simulink model "PMSM_control"  (R2018a)
settings: Solver=VariableStepAuto  StartTime=0.0  StopTime=50  FixedStep=0.0005  MaxStep=0.01
values from neighbouring files (symbols this model uses):
  b_eq = b_m + b_l/r^2    (= 1.5637748692e-05)    [PMSM_AyME.m]    (also in estabilidad_open_loop.m)
  ba = n*J_eq*w_pos    (= 0.0113019895361)    [PMSM_AyME.m]
  C_t = 1.091    [PMSM_AyME.m]
  J_eq = J_m + J_l/r^2    (= 5.65099476805e-06)    [PMSM_AyME.m]    (also in estabilidad_open_loop.m)
  K_e_omega = 3*p_obs^2    (= 30720000)    [PMSM_AyME.m]
  K_e_theta = -3*p_obs    (= 9600)    [PMSM_AyME.m]
  Ksa = n*J_eq*w_pos*w_pos    (= 9.04159162887)    [PMSM_AyME.m]
  Ksia = J_eq*w_pos*w_pos*w_pos    (= 2893.30932124)    [PMSM_AyME.m]
  L_d = 6.6E-3    (= 0.0066)    [PMSM_AyME.m]    (also in estabilidad_open_loop.m)
  L_q = 5.8E-3    (= 0.0058)    [PMSM_AyME.m]    (also in estabilidad_open_loop.m)
  lambda_m = 0.01546    [PMSM_AyME.m]    (also in estabilidad_open_loop.m)
  Lls = 0.8E-3    (= 0.0008)    [PMSM_AyME.m]    (also in estabilidad_open_loop.m)
  Pp = 3    [PMSM_AyME.m]    (also in estabilidad_open_loop.m)
  r = 314.3008    [PMSM_AyME.m]    (also in estabilidad_open_loop.m)
  R_0 = -p_i*Lls    (= 4)    [PMSM_AyME.m]
  R_d = -p_i*L_d    (= 33)    [PMSM_AyME.m]
  R_q = -p_i*L_q    (= 29)    [PMSM_AyME.m]
  R_s = 1.02    [PMSM_AyME.m]    (also in estabilidad_open_loop.m)
  R_tsa = 55    [PMSM_AyME.m]
  Tl = 1.57    [PMSM_AyME.m]    (also in estabilidad_open_loop.m)
undefined symbols (not defined in the file or in its folder): sigbuilder_block
libraries: dspsigops x3, peTransforms x1, simulink x1
settings Model: PacingRate=1000  Creator=gino  LastModifiedBy=gino
settings SolverCC: ZeroCrossControl=EnableAll

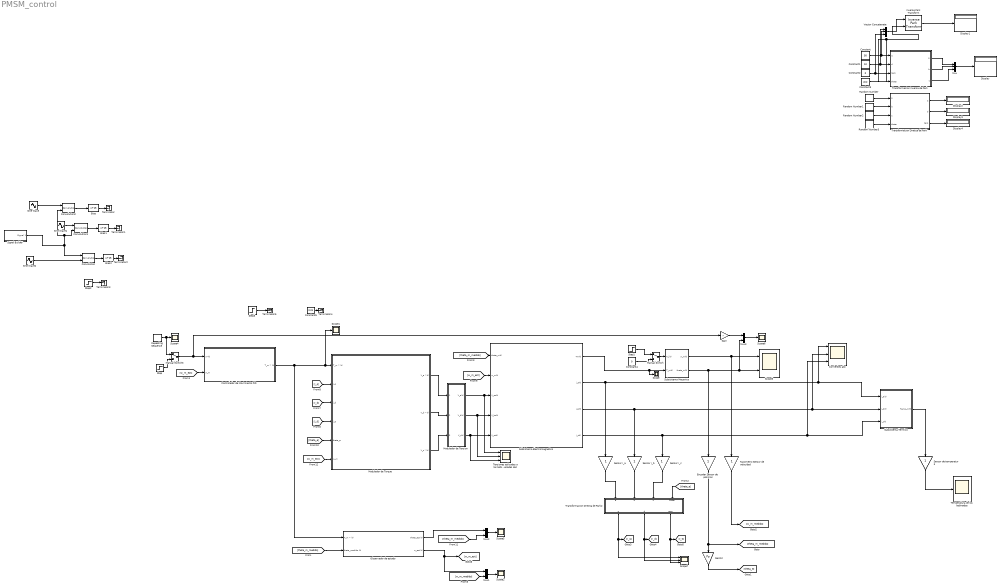
== system PMSM_control ==
  Bias : Bias  Bias=15
  Bias1 : Bias  Bias=15
  Bias2 : Bias  Bias=15
  Constant : Constant  Value=50
  Constant1 : Constant  Value=10
  Constant2 : Constant  Value=0
  Constant3 : Constant  Value=pi/2
  Constant4 : Constant  Value=0
  Constant5 : Constant  Value=0.01
  Controlador de Movimiento PID : Subsystem
  Convolution : dspsigops/Convolution  domain=Time  roundingMode=Floor  overflowMode=off  outputDataTypeStr=Inherit: Same as accumulator  outputMin=[]  outputMax=[]  outputLastDataTypeStr=Inherit: Same as accumulator
      settings: SourceProductName=DSP System Toolbox  SourceProductBaseCode=DS
  Convolution1 : dspsigops/Convolution  domain=Time  roundingMode=Floor  overflowMode=off  outputDataTypeStr=Inherit: Same as accumulator  outputMin=[]  outputMax=[]  outputLastDataTypeStr=Inherit: Same as accumulator
      settings: SourceProductName=DSP System Toolbox  SourceProductBaseCode=DS
  Convolution2 : dspsigops/Convolution  domain=Time  roundingMode=Floor  overflowMode=off  outputDataTypeStr=Inherit: Same as accumulator  outputMin=[]  outputMax=[]  outputLastDataTypeStr=Inherit: Same as accumulator
      settings: SourceProductName=DSP System Toolbox  SourceProductBaseCode=DS
  Corrientes abc : Scope  NumInputPorts=3
  Display{,1..4} (5 alike) : Display
  Encoder Sensor de posicion : Gain
  Gain : Gain  Gain=r
  Gain12 : Gain  Gain=Pp
  Inverse Park Transform : peTransforms/Inverse Park Transform  AxisAlignment=Q-axis  PowerInvariant=off
  Manual Switch : ManualSwitch
  Manual Switch3 : ManualSwitch
  Modulador de Tension : Subsystem
  Modulador de Torque : Subsystem
  Mux : Mux  Inputs=3
  Mux1 : Mux  Inputs=2
  Mux2 : Mux  Inputs=2
  Mux3 : Mux  Inputs=2
  Observador de estado : Subsystem
  Random Number{,1..3} (4 alike) : RandomNumber  SampleTime=0.1
  Repeating Sequence : simulink/Sources/Repeating Sequence  rep_seq_t=[0 5 10 15 20 25 30 35 40]  rep_seq_y="[0 0 2*pi 2*pi 0 0  -2*pi -2*pi 0]"
  Scope{,1..2,4..6} (6 alike) : Scope
  Scope3 : Scope  NumInputPorts=2
  Scope7 : Scope  NumInputPorts=3
  Sensor de temperatura : Gain
  Sensor i_a : Gain
  Sensor i_b : Gain
  Sensor i_c : Gain
  Signal Builder : Subsystem  Tag=STV Subsys  LoadFcn=sigbuilder_block('load');  StartFcn=sigbuilder_block('start');  StopFcn=sigbuilder_block('stop');  ClipboardFcn=sigbuilder_block('clipboard');  mask(Sigbuilder block){tuvar=[0:10]}
      mask help: Simulink:masks:SigbuilderBlock_MD
      mask init:
      | if ~strcmp(get_param(bdroot(gcbh),'SimulationStatus'),'stopped') tuvar = sigbuilder_block('maskInit'); end
      settings: CopyFcn=sigbuilder_block('copy');  DeleteFcn=sigbuilder_block('delete');  ModelCloseFcn=sigbuilder_block('modelClose');  PreSaveFcn=sigbuilder_block('preSave');  PauseFcn=sigbuilder_block('pause');  ContinueFcn=sigbuilder_block('continue');  NameChangeFcn=sigbuilder_block('namechange');  OpenFcn=sigbuilder_block('open',[242.25 102.75 550.5 357 ]);  CloseFcn=sigbuilder_block('close');
      mask Display: plot(0, 0, 100, 100,[2, 2, 32, 32, 2], [68, 8, 8, 68, 68],[32, 2], [38, 38], [32, 19, 2],[53, 60, 44], [32, 17, 17, 2],[16, 16, 31, 31]);txt = getActiveGroup(gcbh);text(2, 100, txt,'verticalAlignment', 'top');
  Sine Wave : Sin  Amplitude=30  Frequency=300*2*pi  SampleTime=0
  Sine Wave1 : Sin  Amplitude=30  Frequency=300*2*pi  Phase=2*pi/3  SampleTime=0
  Sine Wave2 : Sin  Amplitude=30  Frequency=300*2*pi  Phase=4*pi/3  SampleTime=0
  Step : Step  After=0.1  SampleTime=0
  Step1 : Step  Time=0.3  After=Tl  SampleTime=0
  Step2 : Step  Time=0.1  After=19.596  SampleTime=0
  Step3 : Step  Time=0.1  After=0.001  SampleTime=0
  Subsistema Electromagnetico : Subsystem
  Subsistema Mecanico : Subsystem
  Subsistema Termico : Subsystem
  Tacometro Sensor de velocidad : Gain
  Temperatura de los bobinados : Scope
  Tensiones aplicadas a los bobinados en coordenadas abc : Scope  NumInputPorts=3
  Terminator{,1..5} (6 alike) : Terminator
  Transformacion Directa de Park : MATLAB Function  TreatAsAtomicUnit=on
  Transformacion Directa de Park2 : MATLAB Function  TreatAsAtomicUnit=on
  Transformacion Inversa de Park : MATLAB Function  TreatAsAtomicUnit=on
  Vector Concatenate : Concatenate  NumInputs=3
  wires:
  Constant3/1 -> Inverse Park Transform/2, Transformacion Inversa de Park/4(theta)
  Constant2/1 -> Vector Concatenate/3, Transformacion Inversa de Park/3(zero)
  Constant1/1 -> Vector Concatenate/1, Transformacion Inversa de Park/2(d)
  Constant/1 -> Vector Concatenate/2, Transformacion Inversa de Park/1(q)
  Transformacion Inversa de Park/2(b) -> Mux/2
  Transformacion Inversa de Park/1(a) -> Mux/1
  Transformacion Inversa de Park/3(c) -> Mux/3
  Mux/1 -> Display/1
  Vector Concatenate/1 -> Inverse Park Transform/1
  Inverse Park Transform/1 -> Display1/1
  Manual Switch/1 -> Subsistema Mecanico/1(T_l(t))
  Constant4/1 -> Manual Switch/2
  Convolution1/1 -> Bias1/1
  Signal Builder/1(Signal 1) -> Convolution/1, Convolution1/2, Convolution2/2
  Sine Wave2/1 -> Convolution/2
  Sine Wave1/1 -> Convolution1/1
  Sine Wave/1 -> Convolution2/1
  Convolution/1 -> Bias2/1
  Convolution2/1 -> Bias/1
  Random Number2/1 -> Transformacion Directa de Park/3(c)
  Random Number3/1 -> Transformacion Directa de Park/4(theta)
  Random Number1/1 -> Transformacion Directa de Park/2(b)
  Random Number/1 -> Transformacion Directa de Park/1(a)
  Transformacion Directa de Park/3(zero) -> Display4/1
  Transformacion Directa de Park/2(d) -> Display3/1
  Transformacion Directa de Park/1(q) -> Display2/1
  Step1/1 -> Manual Switch/1
  Transformacion Directa de Park2/2(d) -> Scope7/2, [i_d]
  Transformacion Directa de Park2/3(zero) -> [i_0], Scope7/3
  Subsistema Electromagnetico/1(Tm(t)) -> Scope/1, Subsistema Mecanico/2(T_m(t))
  Subsistema Mecanico/2(theta_m(t)) -> Mux3/2, Scope3/2, Encoder Sensor de posicion/1
  Modulador de Tension/3(V_c(t)) -> Subsistema Electromagnetico/5(V_cs(t)), Tensiones aplicadas a los bobinados en coordenadas abc/3
  Modulador de Tension/2(V_b(t)) -> Subsistema Electromagnetico/4(V_bs(t)), Tensiones aplicadas a los bobinados en coordenadas abc/2
  Modulador de Tension/1(V_a(t)) -> Tensiones aplicadas a los bobinados en coordenadas abc/1, Subsistema Electromagnetico/3(V_as(t))
  Transformacion Directa de Park2/1(q) -> [i_q], Scope7/1
  Subsistema Mecanico/1(w_m(t)) -> Scope3/1, Tacometro Sensor de velocidad/1
  Subsistema Electromagnetico/2(i_a(t)) -> Sensor i_a/1, Corrientes abc/1, Subsistema Termico/1(i_a(t))
  Subsistema Termico/1(Temp_m(t)) -> Sensor de temperatura/1
  Subsistema Electromagnetico/3(i_b(t)) -> Subsistema Termico/2(i_b(t)), Corrientes abc/2, Sensor i_b/1
  Sensor de temperatura/1 -> Temperatura de los bobinados/1
  Subsistema Electromagnetico/4(i_c(t)) -> Corrientes abc/3, Subsistema Termico/3(i_c(t)), Sensor i_c/1
  Gain12/1 -> [theta_e]
  [theta_m_medido] -> Subsistema Electromagnetico/1("theta_m(t) ")
  [theta_e] -> Transformacion Directa de Park2/4(theta)
  Encoder Sensor de posicion/1 -> Gain12/1, [theta_m_medido]
  Sensor i_b/1 -> Transformacion Directa de Park2/2(b)
  Sensor i_a/1 -> Transformacion Directa de Park2/1(a)
  Sensor i_c/1 -> Transformacion Directa de Park2/3(c)
  Tacometro Sensor de velocidad/1 -> [w_m_medido]
  [w_m_est] -> Subsistema Electromagnetico/2(w_m(t))
  Bias/1 -> Terminator/1
  Bias1/1 -> Terminator1/1
  Bias2/1 -> Terminator2/1
  Step2/1 -> Terminator3/1
  Constant5/1 -> Terminator4/1
  [w_m_est] -> Modulador de Torque/6("w_m ")
  [theta_e] -> Modulador de Torque/5(theta_e)
  [i_0] -> Modulador de Torque/4(i_0)
  [i_d] -> Modulador de Torque/3(i_d)
  [i_q] -> Modulador de Torque/2(i_q)
  Modulador de Torque/3(V_c * (t)) -> Modulador de Tension/3(V_c * (t))
  Modulador de Torque/2(V_b * (t)) -> Modulador de Tension/2(V_b * (t))
  Modulador de Torque/1(V_a * (t)) -> Modulador de Tension/1(V_a * (t))
  Controlador de Movimiento PID/1(T_m *' (t)) -> Scope1/1, Modulador de Torque/1(T_m *' (t)), Observador de estado/1(T_m *' (t))
  Repeating Sequence/1 -> Manual Switch3/1, Scope4/1
  Step/1 -> Manual Switch3/2
  Manual Switch3/1 -> Gain/1, Controlador de Movimiento PID/1(w*(t))
  [w_m_est] -> Controlador de Movimiento PID/2(w_m)
  [theta_m_medido] -> Observador de estado/2(theta_medido (t))
  [w_m_medido] -> Mux1/2
  Observador de estado/2(w_est (t)) -> Mux1/1, [w_m_est]
  Mux1/1 -> Scope2/1
  Mux2/1 -> Scope5/1
  [theta_m_medido] -> Mux2/2
  Observador de estado/1(theta_est (t)) -> Mux2/1
  Step3/1 -> Terminator5/1
  Mux3/1 -> Scope6/1
  Gain/1 -> Mux3/1

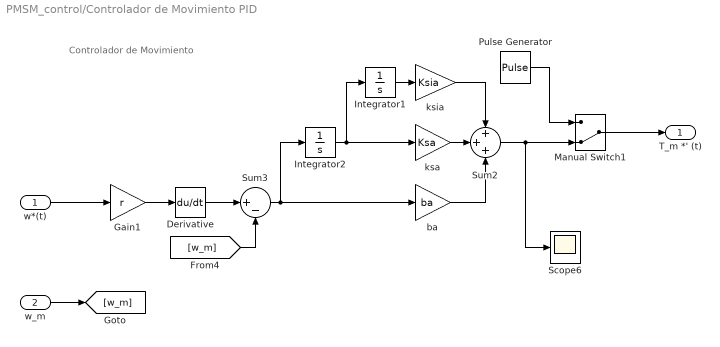
== system PMSM_control/Controlador de Movimiento PID ==
  note: Controlador de Movimiento
  w*(t) : Inport
  w_m : Inport  Port=2
  Derivative : Derivative
  Gain1 : Gain  Gain=r
  Integrator1 : Integrator
  Integrator2 : Integrator
  Manual Switch1 : ManualSwitch  CurrentSetting=0
  Pulse Generator : DiscretePulseGenerator  PulseType=Time based  Amplitude=0.001  Period=1
  Scope6 : Scope
  Sum2 : Sum  Inputs=+++
  Sum3 : Sum  Inputs=|+-
  ba : Gain  Gain=ba
  "ksa " : Gain  Gain=Ksa
  "ksia " : Gain  Gain=Ksia
  T_m *' (t) : Outport
  wires:
  "ksia "/1 -> Sum2/1
  "ksa "/1 -> Sum2/2
  [w_m] -> Sum3/2
  Sum2/1 -> Manual Switch1/2, Scope6/1
  Pulse Generator/1 -> Manual Switch1/1
  Gain1/1 -> Derivative/1
  Integrator2/1 -> "ksa "/1, Integrator1/1
  Integrator1/1 -> "ksia "/1
  Manual Switch1/1 -> T_m *' (t)/1
  Derivative/1 -> Sum3/1
  Sum3/1 -> ba/1, Integrator2/1
  ba/1 -> Sum2/3
  w*(t)/1 -> Gain1/1
  w_m/1 -> [w_m]

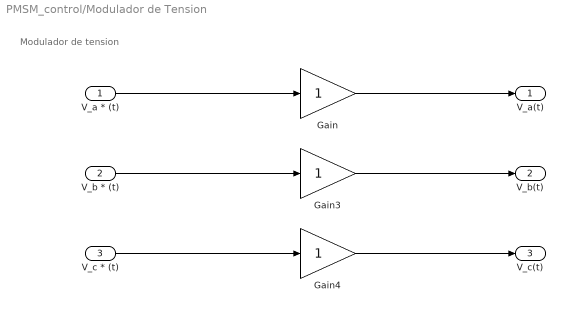
== system PMSM_control/Modulador de Tension ==
  note: Modulador de tension
  V_a * (t) : Inport
  V_b * (t) : Inport  Port=2
  V_c * (t) : Inport  Port=3
  Gain : Gain
  Gain3 : Gain
  Gain4 : Gain
  V_a(t) : Outport
  V_b(t) : Outport  Port=2
  V_c(t) : Outport  Port=3
  wires:
  V_a * (t)/1 -> Gain/1
  Gain/1 -> V_a(t)/1
  V_b * (t)/1 -> Gain3/1
  V_c * (t)/1 -> Gain4/1
  Gain3/1 -> V_b(t)/1
  Gain4/1 -> V_c(t)/1

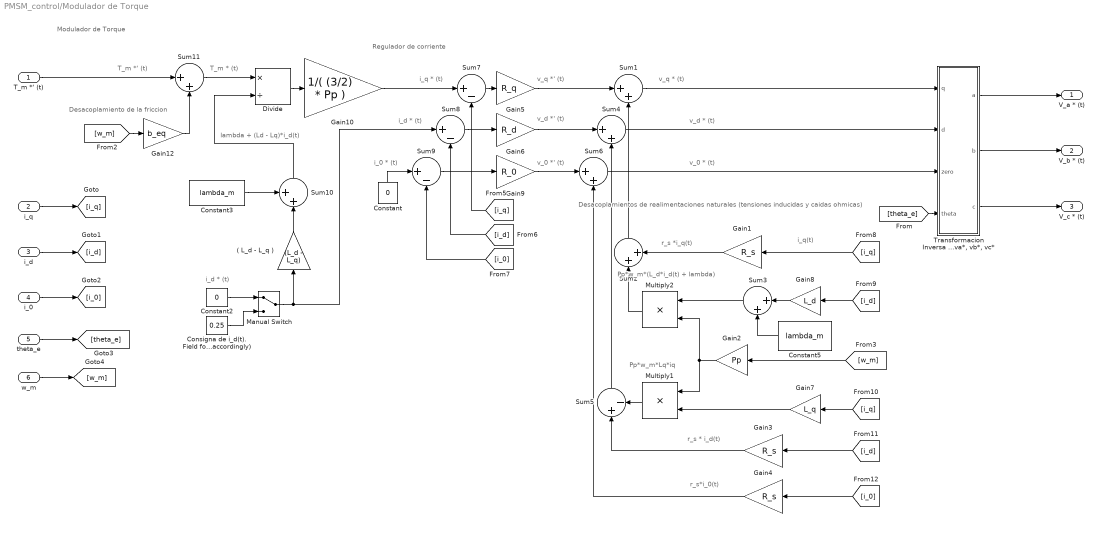
== system PMSM_control/Modulador de Torque ==
  note: lambda + (Ld - Lq)*i_d(t)
  note: Modulador de Torque
  note: T_m *' (t)
  note: Regulador de corriente
  note: Desacoplamiento de la friccion
  note: T_m * (t)
  note: i_d * (t)
  note: i_0 * (t)
  note: i_q * (t)
  note: i_d * (t)
  note: Desacoplamientos de realimentaciones naturales
      | (tensiones inducidas y caidas ohmicas)
  note: v_0 * (t)
  note: v_d * (t)
  note: r_s*i_0(t)
  note: Pp*w_m*Lq*iq
  note: r_s * i_d(t)
  note: Pp*w_m*(L_d*i_d(t) + lambda)
  note: r_s *i_q(t)
  note: v_q * (t)
  note: i_q(t)
  note: v_q *' (t)
  note: v_d *' (t)
  note: v_0 *' (t)
  T_m *' (t) : Inport
  i_q : Inport  Port=2
  i_d : Inport  Port=3
  i_0 : Inport  Port=4
  theta_e : Inport  Port=5
  "w_m " : Inport  Port=6
  ( L_d - L_q ) : Gain  Gain=(L_d - L_q)
  Consigna de i_d(t). Field forcing or weakening (change sign accordingly) : Constant  Value=0.25
  Constant : Constant  Value=0
  Constant2 : Constant  Value=0
  Constant3 : Constant  Value=lambda_m
  Constant5 : Constant  Value=lambda_m
  Divide : Product  Inputs=*/
  Gain1 : Gain  Gain=R_s
  Gain10 : Gain  Gain=1/( (3/2) * Pp )
  Gain12 : Gain  Gain=b_eq
  Gain2 : Gain  Gain=Pp
  Gain3 : Gain  Gain=R_s
  Gain4 : Gain  Gain=R_s
  Gain5 : Gain  Gain=R_q
  Gain6 : Gain  Gain=R_d
  Gain7 : Gain  Gain=L_q
  Gain8 : Gain  Gain=L_d
  Gain9 : Gain  Gain=R_0
  Manual Switch : ManualSwitch
  Multiply1 : Product
  Multiply2 : Product
  Sum{1..4,6,11} (6 alike) : Sum  Inputs=|++
  Sum10 : Sum  Inputs=++|
  Sum{5,7..9} (4 alike) : Sum  Inputs=|+-
  "Transformacion Inversa de Park vq*, vd*, v0* --> va*, vb*, vc*" : MATLAB Function  TreatAsAtomicUnit=on
  V_a * (t) : Outport
  V_b * (t) : Outport  Port=2
  V_c * (t) : Outport  Port=3
  wires:
  Gain7/1 -> Multiply1/2
  [i_q] -> Sum7/2
  Gain5/1 -> Sum1/1
  Sum9/1 -> Gain9/1
  Sum8/1 -> Gain6/1
  Constant5/1 -> Sum3/2
  Sum1/1 -> "Transformacion Inversa de Park vq*, vd*, v0* --> va*, vb*, vc*"/1(q)
  Constant/1 -> Sum9/1
  Sum5/1 -> Sum4/2
  [i_q] -> Gain1/1
  Sum3/1 -> Multiply2/1
  Gain1/1 -> Sum2/2
  [i_0] -> Gain4/1
  Gain2/1 -> Multiply1/1, Multiply2/2
  [i_q] -> Gain7/1
  [i_d] -> Gain3/1
  Sum2/1 -> Sum1/2
  [theta_e] -> "Transformacion Inversa de Park vq*, vd*, v0* --> va*, vb*, vc*"/4(theta)
  Sum6/1 -> "Transformacion Inversa de Park vq*, vd*, v0* --> va*, vb*, vc*"/3(zero)
  Sum4/1 -> "Transformacion Inversa de Park vq*, vd*, v0* --> va*, vb*, vc*"/2(d)
  [i_d] -> Sum8/2
  [i_d] -> Gain8/1
  Gain3/1 -> Sum5/1
  Gain9/1 -> Sum6/1
  [i_0] -> Sum9/2
  Multiply1/1 -> Sum5/2
  Gain6/1 -> Sum4/1
  Sum7/1 -> Gain5/1
  Multiply2/1 -> Sum2/1
  Gain8/1 -> Sum3/1
  Gain4/1 -> Sum6/2
  [w_m] -> Gain2/1
  Constant2/1 -> Manual Switch/1
  Consigna de i_d(t). Field forcing or weakening (change sign accordingly)/1 -> Manual Switch/2
  Gain10/1 -> Sum7/1
  Divide/1 -> Gain10/1
  Constant3/1 -> Sum10/1
  ( L_d - L_q )/1 -> Sum10/2
  Sum10/1 -> Divide/2
  [w_m] -> Gain12/1
  Sum11/1 -> Divide/1
  theta_e/1 -> [theta_e]
  i_q/1 -> [i_q]
  i_0/1 -> [i_0]
  "w_m "/1 -> [w_m]
  i_d/1 -> [i_d]
  T_m *' (t)/1 -> Sum11/1
  Gain12/1 -> Sum11/2
  "Transformacion Inversa de Park vq*, vd*, v0* --> va*, vb*, vc*"/3(c) -> V_c * (t)/1
  "Transformacion Inversa de Park vq*, vd*, v0* --> va*, vb*, vc*"/2(b) -> V_b * (t)/1
  "Transformacion Inversa de Park vq*, vd*, v0* --> va*, vb*, vc*"/1(a) -> V_a * (t)/1
  Manual Switch/1 -> Sum8/1, ( L_d - L_q )/1

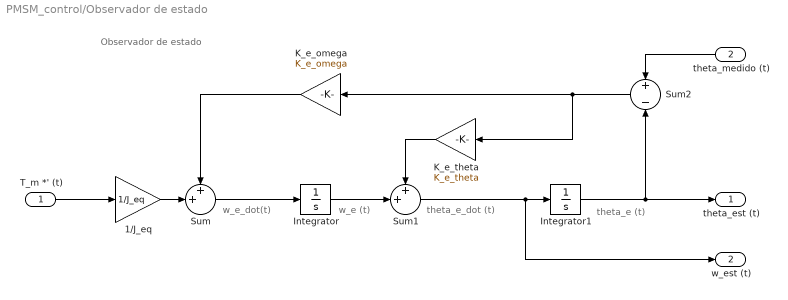
== system PMSM_control/Observador de estado ==
  note: Observador de estado
  note: theta_e (t)
  note: theta_e_dot (t)
  note: w_e (t)
  note: w_e_dot(t)
  T_m *' (t) : Inport
  theta_medido (t) : Inport  Port=2
  1/J_eq : Gain  Gain=1/J_eq
  Integrator : Integrator
  Integrator1 : Integrator
  K_e_omega : Gain  Gain=K_e_omega
  K_e_theta : Gain  Gain=K_e_theta
  Sum : Sum  Inputs=++|
  Sum1 : Sum  Inputs=++|
  Sum2 : Sum  Inputs=+-
  theta_est (t) : Outport
  w_est (t) : Outport  Port=2
  wires:
  Integrator1/1 -> theta_est (t)/1, Sum2/2
  Sum/1 -> Integrator/1
  T_m *' (t)/1 -> 1/J_eq/1
  1/J_eq/1 -> Sum/2
  K_e_omega/1 -> Sum/1
  Integrator/1 -> Sum1/2
  K_e_theta/1 -> Sum1/1
  Sum1/1 -> w_est (t)/1, Integrator1/1
  theta_medido (t)/1 -> Sum2/1
  Sum2/1 -> K_e_theta/1, K_e_omega/1

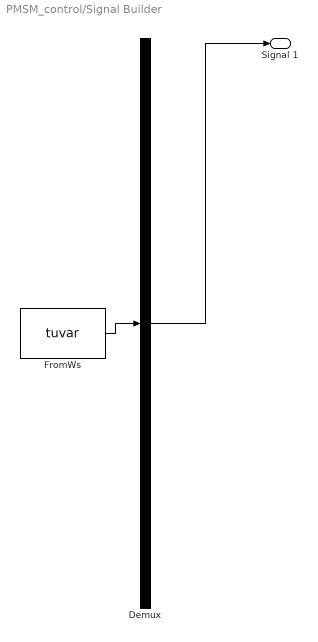
== system PMSM_control/Signal Builder ==
  Demux : Demux  Tag=STV Demux  Outputs=1
  FromWs : FromWorkspace  Tag=STV FromWs  VariableName=tuvar  SampleTime=0
      SigBuilderData=|
      | common.afterFinalStr = 'Extrapolate'
      | common.sampleTime = 0
      | dataSet.timeRange = [0 10]
      | dataSet.name = 'Group 1'
      | sbobj.Groups.Name = 'Group 1'
      | sbobj.Groups.Signals.Name = 'Signal 1'
      | sbobj.Groups.Signals.XData = [0 0.49 10]
      | sbobj.Groups.Signals.YData = [0 1 1]
  Signal 1 : Outport  Tag=STV Outport
  wires:
  Demux/1 -> Signal 1/1
  FromWs/1 -> Demux/1

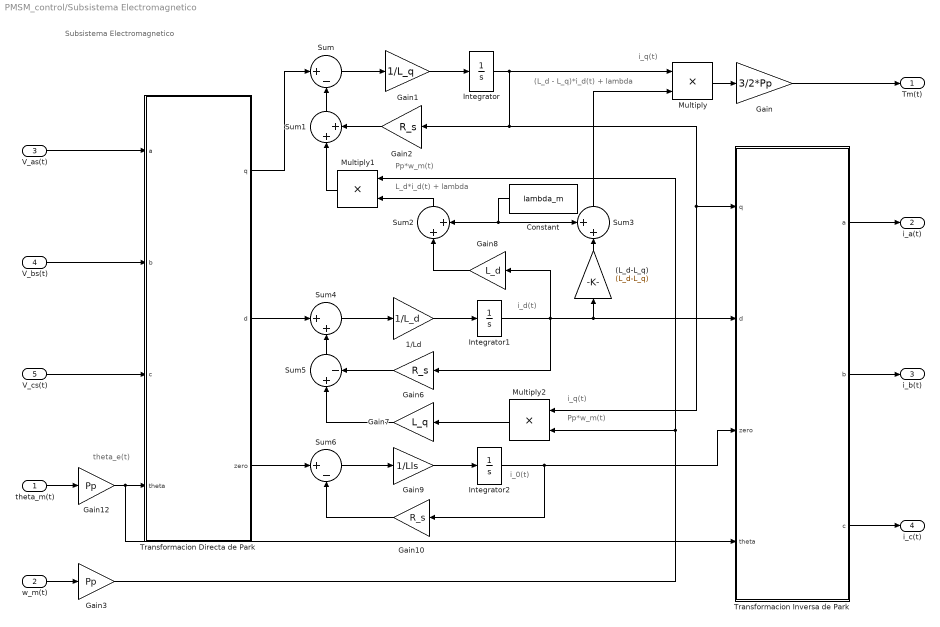
== system PMSM_control/Subsistema Electromagnetico ==
  note: Subsistema Electromagnetico
  note: (L_d - L_q)*i_d(t) + lambda
  note: L_d*i_d(t) + lambda
  note: theta_e(t)
  note: i_0(t)
  note: Pp*w_m(t)
  note: Pp*w_m(t)
  note: i_q(t)
  note: i_d(t)
  note: i_q(t)
  "theta_m(t) " : Inport
  w_m(t) : Inport  Port=2
  V_as(t) : Inport  Port=3
  V_bs(t) : Inport  Port=4
  V_cs(t) : Inport  Port=5
  (L_d-L_q) : Gain  Gain=(L_d-L_q)
  1/Ld : Gain  Gain=1/L_d
  Constant : Constant  Value=lambda_m
  Gain : Gain  Gain=3/2*Pp
  Gain1 : Gain  Gain=1/L_q
  Gain10 : Gain  Gain=R_s
  Gain12 : Gain  Gain=Pp
  Gain2 : Gain  Gain=R_s
  Gain3 : Gain  Gain=Pp
  Gain6 : Gain  Gain=R_s
  Gain7 : Gain  Gain=L_q
  Gain8 : Gain  Gain=L_d
  Gain9 : Gain  Gain=1/Lls
  Integrator : Integrator
  Integrator1 : Integrator
  Integrator2 : Integrator
  Multiply : Product
  Multiply1 : Product
  Multiply2 : Product
  Sum : Sum  Inputs=|+-
  Sum1 : Sum  Inputs=|++
  Sum2 : Sum  Inputs=|++
  Sum3 : Sum  Inputs=++|
  Sum4 : Sum  Inputs=|++
  Sum5 : Sum  Inputs=|+-
  Sum6 : Sum  Inputs=|+-
  Transformacion Directa de Park : MATLAB Function  TreatAsAtomicUnit=on
  Transformacion Inversa de Park : MATLAB Function  TreatAsAtomicUnit=on
  Tm(t) : Outport
  i_a(t) : Outport  Port=2
  i_b(t) : Outport  Port=3
  i_c(t) : Outport  Port=4
  wires:
  Gain/1 -> Tm(t)/1
  Multiply/1 -> Gain/1
  Integrator/1 -> Multiply/1, Transformacion Inversa de Park/1(q), Multiply2/1, Gain2/1
  Gain1/1 -> Integrator/1
  Sum/1 -> Gain1/1
  Sum1/1 -> Sum/2
  Gain2/1 -> Sum1/2
  Multiply1/1 -> Sum1/1
  w_m(t)/1 -> Gain3/1
  Gain3/1 -> Multiply1/1, Multiply2/2
  Sum3/1 -> Multiply/2
  Constant/1 -> Sum3/1, Sum2/2
  (L_d-L_q)/1 -> Sum3/2
  Integrator1/1 -> Gain6/1, Transformacion Inversa de Park/2(d), (L_d-L_q)/1, Gain8/1
  1/Ld/1 -> Integrator1/1
  Sum4/1 -> 1/Ld/1
  Gain6/1 -> Sum5/2
  Gain7/1 -> Sum5/1
  Multiply2/1 -> Gain7/1
  Gain8/1 -> Sum2/1
  Sum5/1 -> Sum4/2
  Transformacion Directa de Park/1(q) -> Sum/1
  Transformacion Directa de Park/2(d) -> Sum4/1
  Gain9/1 -> Integrator2/1
  Sum6/1 -> Gain9/1
  Gain10/1 -> Sum6/2
  Integrator2/1 -> Gain10/1, Transformacion Inversa de Park/3(zero)
  Transformacion Directa de Park/3(zero) -> Sum6/1
  "theta_m(t) "/1 -> Gain12/1
  Gain12/1 -> Transformacion Directa de Park/4(theta), Transformacion Inversa de Park/4(theta)
  V_as(t)/1 -> Transformacion Directa de Park/1(a)
  V_bs(t)/1 -> Transformacion Directa de Park/2(b)
  V_cs(t)/1 -> Transformacion Directa de Park/3(c)
  Transformacion Inversa de Park/1(a) -> i_a(t)/1
  Transformacion Inversa de Park/2(b) -> i_b(t)/1
  Transformacion Inversa de Park/3(c) -> i_c(t)/1
  Sum2/1 -> Multiply1/2

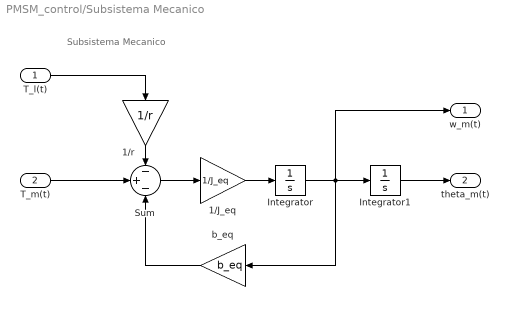
== system PMSM_control/Subsistema Mecanico ==
  note: Subsistema Mecanico
  T_l(t) : Inport
  T_m(t) : Inport  Port=2
  1/J_eq : Gain  Gain=1/J_eq
  1/r : Gain  Gain=1/r
  Integrator : Integrator
  Integrator1 : Integrator
  Sum : Sum  Inputs=-+-
  b_eq : Gain  Gain=b_eq
  w_m(t) : Outport
  theta_m(t) : Outport  Port=2
  wires:
  1/J_eq/1 -> Integrator/1
  Integrator1/1 -> theta_m(t)/1
  Integrator/1 -> Integrator1/1, w_m(t)/1, b_eq/1
  Sum/1 -> 1/J_eq/1
  T_l(t)/1 -> 1/r/1
  b_eq/1 -> Sum/3
  T_m(t)/1 -> Sum/2
  1/r/1 -> Sum/1

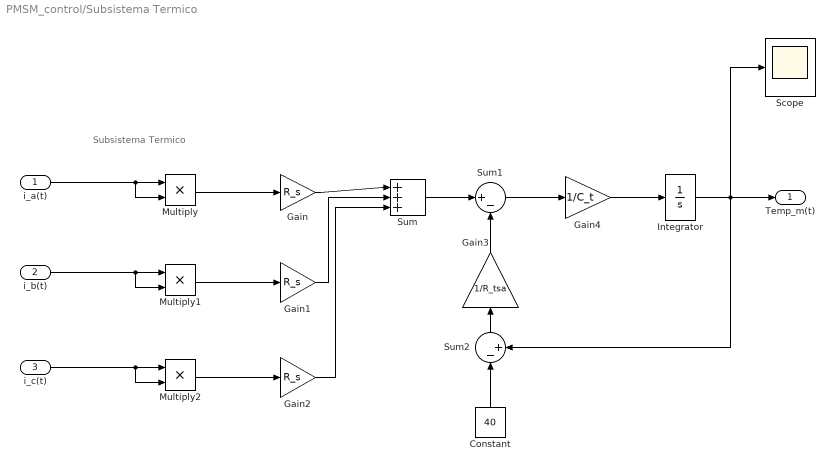
== system PMSM_control/Subsistema Termico ==
  note: Subsistema Termico
  i_a(t) : Inport
  i_b(t) : Inport  Port=2
  i_c(t) : Inport  Port=3
  Constant : Constant  Value=40
  Gain : Gain  Gain=R_s
  Gain1 : Gain  Gain=R_s
  Gain2 : Gain  Gain=R_s
  Gain3 : Gain  Gain=1/R_tsa
  Gain4 : Gain  Gain=1/C_t
  Integrator : Integrator  InitialCondition=40
  Multiply : Product
  Multiply1 : Product
  Multiply2 : Product
  Scope : Scope
  Sum : Sum  Inputs=|+++
  Sum1 : Sum  Inputs=|+-
  Sum2 : Sum  Inputs=|-+
  Temp_m(t) : Outport
  wires:
  i_a(t)/1 -> Multiply/1, Multiply/2
  i_b(t)/1 -> Multiply1/2, Multiply1/1
  i_c(t)/1 -> Multiply2/2, Multiply2/1
  Multiply/1 -> Gain/1
  Multiply1/1 -> Gain1/1
  Multiply2/1 -> Gain2/1
  Gain1/1 -> Sum/2
  Gain/1 -> Sum/1
  Gain2/1 -> Sum/3
  Sum/1 -> Sum1/1
  Gain3/1 -> Sum1/2
  Sum2/1 -> Gain3/1
  Constant/1 -> Sum2/1
  Sum1/1 -> Gain4/1
  Gain4/1 -> Integrator/1
  Integrator/1 -> Sum2/2, Temp_m(t)/1, Scope/1

== matlab function PMSM_control/Transformacion Inversa de Park ==
  data: q input; a output; d input; zero input; theta input; b output; c output
function [a, b, c] = inverse_park_transformation(q, d, zero, theta)
%Transformación inversa de Park
 
abc = [cos(theta)               sin(theta)              1
        cos(theta - 2*pi/3)     sin(theta - 2*pi/3)     1
        cos(theta + 2*pi/3)     sin(theta + 2*pi/3)     1] ...
    *   [q
        d
        zero];

a = abc(1);
b = abc(2);
c = abc(3);

end

== matlab function PMSM_control/Transformacion Directa de Park ==
  data: a input; q output; b input; c input; theta input; d output; zero output
function [q, d, zero] = park_transformation(a, b, c, theta)
%Transformación directa de Park
 
qdz = 2/3 * [cos(theta)     cos(theta - 2*pi/3)     cos(theta + 2*pi/3)
                    sin(theta)      sin(theta - 2*pi/3)     sin(theta + 2*pi/3)
                    1/2             1/2                     1/2] ...
                *   [a
                    b 
                    c];

q = qdz(1);
d = qdz(2);
zero = qdz(3);

end

== matlab function PMSM_control/Subsistema Electromagnetico/Transformacion Directa de Park ==
  data: a input; q output; b input; c input; theta input; d output; zero output
function [q, d, zero] = park_transformation(a, b, c, theta)
%Transformación directa de Park
 
qdz = 2/3 * [cos(theta)     cos(theta - 2*pi/3)     cos(theta + 2*pi/3)
                    sin(theta)      sin(theta - 2*pi/3)     sin(theta + 2*pi/3)
                    1/2             1/2                     1/2] ...
                *   [a
                    b 
                    c];

q = qdz(1);
d = qdz(2);
zero = qdz(3);

end

== matlab function PMSM_control/Subsistema Electromagnetico/Transformacion Inversa de Park ==
  data: q input; a output; d input; zero input; theta input; b output; c output
function [a, b, c] = inverse_park_transformation(q, d, zero, theta)
%Transformación inversa de Park
 
abc = [cos(theta)               sin(theta)              1
        cos(theta - 2*pi/3)     sin(theta - 2*pi/3)     1
        cos(theta + 2*pi/3)     sin(theta + 2*pi/3)     1] ...
    *   [q
        d
        zero];

a = abc(1);
b = abc(2);
c = abc(3);

end

== matlab function PMSM_control/Modulador de Torque/Transformacion Inversa de Park vq*, vd*, v0* --> va*, vb*, vc* ==
  data: q input; a output; d input; zero input; theta input; b output; c output
function [a, b, c] = inverse_park_transformation(q, d, zero, theta)
%Transformación inversa de Park
 
abc = [cos(theta)               sin(theta)              1
        cos(theta - 2*pi/3)     sin(theta - 2*pi/3)     1
        cos(theta + 2*pi/3)     sin(theta + 2*pi/3)     1] ...
    *   [q
        d
        zero];

a = abc(1);
b = abc(2);
c = abc(3);

end

== matlab function PMSM_control/Transformacion Directa de Park2 ==
  data: a input; q output; b input; c input; theta input; d output; zero output
function [q, d, zero] = park_transformation(a, b, c, theta)
%Transformación directa de Park
 
qdz = 2/3 * [cos(theta)     cos(theta - 2*pi/3)     cos(theta + 2*pi/3)
                    sin(theta)      sin(theta - 2*pi/3)     sin(theta + 2*pi/3)
                    1/2             1/2                     1/2] ...
                *   [a
                    b 
                    c];

q = qdz(1);
d = qdz(2);
zero = qdz(3);

end
